simulink model "model_simulation"  (R2018b)
settings: Solver=VariableStepAuto  StartTime=0.0  StopTime=10.0  RelTol=1e-3
undefined symbols (not defined in the file or in its folder): Ts
settings Model: Creator=Alireza  LastModifiedBy=Alireza

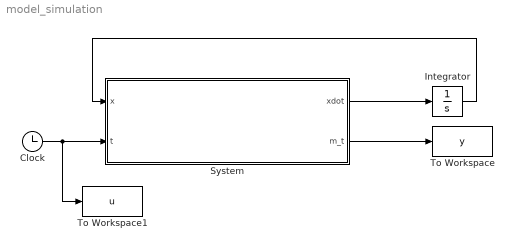
== system model_simulation ==
  Clock : Clock
  Integrator : Integrator
  System : MATLAB Function  TreatAsAtomicUnit=on
  To Workspace : ToWorkspace  VariableName=y  SampleTime=Ts
      settings: Save2DSignal=2-D array (concatenate along first dimension)
  To Workspace1 : ToWorkspace  VariableName=u  SampleTime=Ts
      settings: Save2DSignal=2-D array (concatenate along first dimension)
  wires:
  System/1(xdot) -> Integrator/1
  Integrator/1 -> System/1(x)
  Clock/1 -> To Workspace1/1, System/2(t)
  System/2(m_t) -> To Workspace/1

== matlab function model_simulation/System ==
  data: x input; xdot output; t input; m_t output
function [xdot, m_t] = fcn(x, t)

m_t = 10*sin(0.5*t)+cos(t);
xdot = ((100/(150+m_t))*2*sin(t))-0.5*x^3*(0.3/(150+m_t));
